simulink model "workspace_test"  (R2020b)
settings: Solver=VariableStepAuto  StartTime=0.0  StopTime=10.0  RelTol=1e-3
settings Model: Creator=Rick  LastModifiedBy=Rick

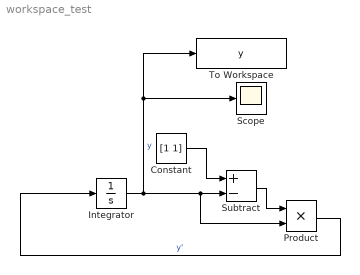
== system workspace_test ==
  Constant : Constant  Value=[1 1]
  Integrator : Integrator  InitialCondition=[0.5 0.6]
  Product : Product
  Scope : Scope
  Subtract : Sum  Inputs=+-
  To Workspace : ToWorkspace  VariableName=y  SampleTime=-1
      settings: MaxDataPoints=1
  wires:
  Product/1 -> Integrator/1  "y'"
  Integrator/1 -> To Workspace/1, Scope/1, Product/2, Subtract/2  "y"
  Constant/1 -> Subtract/1
  Subtract/1 -> Product/1
